simulink model "Longitudinal"  (R2024b)
settings: Solver=VariableStepAuto  StartTime=0.0  StopTime=10.0  RelTol=1e-3
settings Model: Creator=GH-X-ST  LastModifiedBy=GH-X-ST

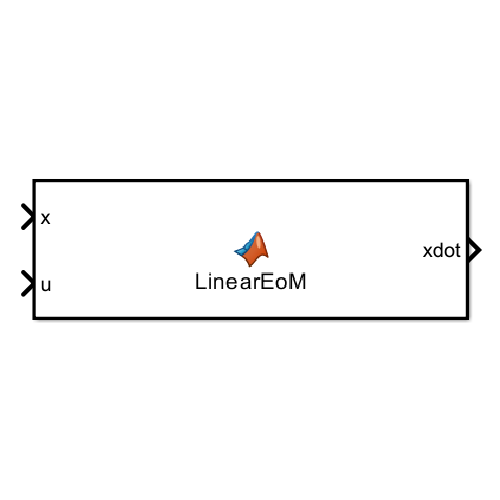
[thumbnail: Simulink's stored preview of the top-level diagram]
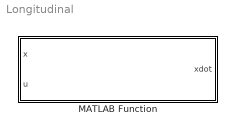
== system Longitudinal ==
  MATLAB Function : MATLAB Function  TreatAsAtomicUnit=on

== matlab function Longitudinal/MATLAB Function ==
  data: x input; u input; xdot output
function xdot = LinearEoM(x,u)
%Input:  - x:Longitudinal state vactor (5x1 vector)
%          x(1)- u      m/s
%          x(2)- w      m/s
%          x(3)- q      rad/s
%          x(4)- theta  rad
%          x(5)- height m
%
%        - u: longitudinal control vector (2x1 vector)
%          u(1)- elevator deflection as percentage of max +ve defrlaction
%               -2<u(1)<1     
%          u(2)- Thrust as % of max thrust
%
%Output: - xdot: (5x1 vector)

% Please open the Preparatory.mlx for matrix construction
Long = load("Long.mat");

A = Long.A_long;

B = Long.B_long;

u(1) = u(1) * 5 * pi / 180; % Elevator(5 deg per step) deflection (rad)

xdot = A*x + B*u;           % Output
